simulink model "Transmitt_Receive_Running_CPU1"  (R2020a)
settings: Solver=FixedStepDiscrete  StartTime=0.0  StopTime=Inf  FixedStep=0.01  RelTol=1e-3  EnableMultiTasking=on
libraries: c280xlib x2, c2000lib x1
settings Model: ExtModeTrigDuration=8  Creator=User-1  LastModifiedBy=NRPU
settings OptimizationCC: DefaultUnderspecifiedDataType=single  EnhancedBackFolding=on  PassReuseOutputArgsAs=Individual arguments  MaxStackSize=1024  OptimizeBlockOrder=speed  DifferentSizesBufferReuse=on  OptimizationCustomize=off  DenormalBehavior=FlushToZero  EfficientTunableParamExpr=on
settings DebuggingCC: ParameterTunabilityLossMsg=error
settings HardwareCC: ProdBitPerChar=16  ProdBitPerInt=16  ProdBitPerPointer=32  ProdBitPerSizeT=32  ProdBitPerPtrDiffT=32  ProdLargestAtomicInteger=Integer  ProdLargestAtomicFloat=None  ProdWordSize=16  ProdLongLongMode=on  ProdHWDeviceType=Texas Instruments->C2000
settings SFSimCC: MATLABDynamicMemAlloc=off
settings RTWCC: SystemTargetFile=ert.tlc  HardwareBoard=TI Delfino F28379D LaunchPad  TLCOptions=-aInlineSetEventsForThisBaseRateFcn=TLC_FALSE -aSuppressMultiTaskScheduler=TLC_FALSE -aRateBasedStepFcn=1  TemplateMakefile=ert_default_tmf  Toolchain=Texas Instruments Code Composer Studio (C2000)
settings CodeAppCC: ForceParamTrailComments=on  IgnoreCustomStorageClasses=off  OperatorAnnotations=on  SimulinkDataObjDesc=on  SFDataObjDesc=on  InsertBlockDesc=on
settings ERTTargetCC: CodeReplacementLibrary=TI C28x  ExtModeStaticAllocSize=10000

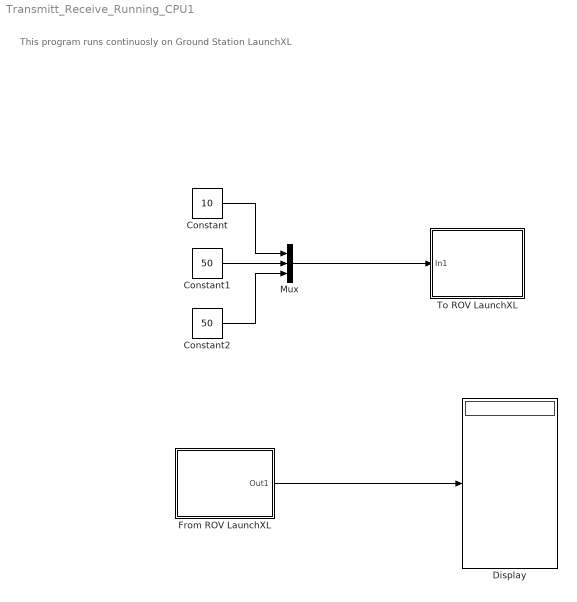
== system Transmitt_Receive_Running_CPU1 ==
  note: This program runs continuosly on Ground Station LaunchXL
  Constant : Constant  Value=10  OutDataTypeStr=single
  Constant1 : Constant  Value=50  OutDataTypeStr=single
  Constant2 : Constant  Value=50  OutDataTypeStr=single
  Display : Display
  From ROV LaunchXL : Subsystem
  Mux : Mux  Inputs=3
  To ROV LaunchXL : Subsystem
  wires:
  Constant1/1 -> Mux/2
  Constant/1 -> Mux/1
  Constant2/1 -> Mux/3
  Mux/1 -> To ROV LaunchXL/1(In1)
  From ROV LaunchXL/1(Out1) -> Display/1

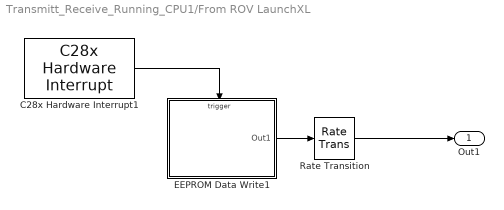
== system Transmitt_Receive_Running_CPU1/From ROV LaunchXL ==
  C28x Hardware Interrupt1 : c2000lib/Scheduling/C28x Hardware Interrupt  irqnumbers=9  pienumbers=3  irqpriorities=30  irqpreempts=1  showinput=off  dspchiptype=C280X
      settings: SourceProductBaseCode=TIC2000
  EEPROM Data Write1 : Subsystem  TreatAsAtomicUnit=on
  Rate Transition : RateTransition  Integrity=off
  Out1 : Outport
  wires:
  EEPROM Data Write1/1(Out1) -> Rate Transition/1
  C28x Hardware Interrupt1/1 -> EEPROM Data Write1/Trigger
  Rate Transition/1 -> Out1/1

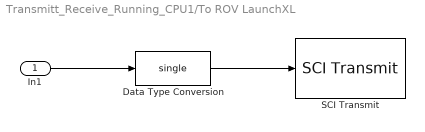
== system Transmitt_Receive_Running_CPU1/To ROV LaunchXL ==
  In1 : Inport
  Data Type Conversion : DataTypeConversion  OutDataTypeStr=single
  SCI Transmit : c280xlib/SCI Transmit  sciModule=B  dataHead='S'  dataTail='E'  postInterrupt=on  numFifo=3
  wires:
  Data Type Conversion/1 -> SCI Transmit/1
  In1/1 -> Data Type Conversion/1

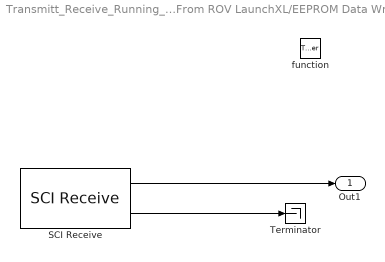
== system Transmitt_Receive_Running_CPU1/From ROV LaunchXL/EEPROM Data Write1 ==
  function : TriggerPort  TriggerType=function-call  VariantControl=Variant
  SCI Receive : c280xlib/SCI Receive  sciModule=B  dataHead='S'  dataTail='E'  dataType=single  dataDim=4  initValue=0  errOption=Output the last received value  errValue=0  sampleTime=-1  outputStatus=on  postInterrupt=on  numFifo=4
      settings: SourceProductBaseCode=TIC2000
  Terminator : Terminator
  Out1 : Outport
  wires:
  SCI Receive/1 -> Out1/1
  SCI Receive/2 -> Terminator/1
